simulink model "Autopilot_Controllers"  (R2020a)
settings: Solver=FixedStepAuto  StartTime=0.0  StopTime=10.0  FixedStep=0.01  RelTol=1e-3
model workspace: external: MAT-File E:\Autopilot\Task 7\GP04_Task7_Codes\JETSTAR_FC4_Parameters.mat (data not in the file)
values from neighbouring files (symbols this model uses):
  g = 32.17405    [JETSTAR_FC4_Parameters.mat]    (also in ReadExcelModified.m = aircraft_data(52))
  u_0 = 585.349466728    [JETSTAR_FC4_Parameters.mat]    (also in ReadExcelModified.m = s0(1))
settings Model: Creator=mohan  LastModifiedBy=mohan

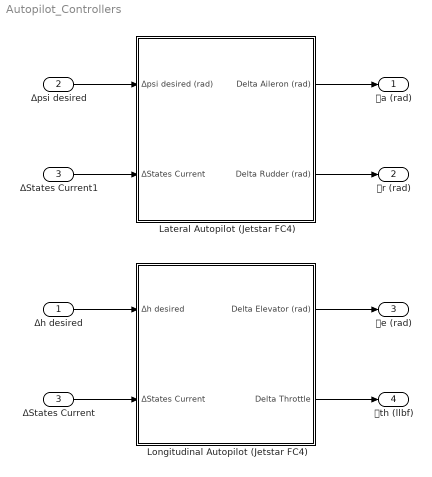
== system Autopilot_Controllers ==
  Δh desired : Inport
  Δpsi desired : Inport  Port=2
  ΔStates Current : Inport  Port=3
  Lateral Autopilot (Jetstar FC4) : Subsystem  mask{Kp_yaw=0.38326, taw_HPF=1/0.7, Kp_roll=1.0063, Kd_roll=0.32967, taw_coordination=20}
      mask prompts: Kp_yaw "Kp"; taw_HPF "Taw (Washout)"; Kp_roll "Kp"; Kd_roll "Kd"; taw_coordination "Taw"
      mask DialogControl ParameterGroupVar Prompt: Controllers
      mask DialogControl Container4 Prompt: Yaw Damper Gains (P + Washout)
      mask DialogControl Container5 Prompt: Roll Controller (PD)
      mask DialogControl Container6 Prompt: Coordinated Turn
  Longitudinal Autopilot (Jetstar FC4) : Subsystem  mask{Kp_alt=0.001862, Kd_alt=0.001694, Kp_pitch=1.6546, a_pitch=0.4868, Kd_pitch=0.52894, Kp_vel=1027.7, a_vel=0.05, Kd_vel=1523.9, zero_vel=0.1, pole_vel=0.7033}
      mask prompts: Kp_alt "Kp"; Kd_alt "Kd"; Kp_pitch "Kp"; a_pitch "a"; Kd_pitch "Kd"; Kp_vel "Kp"; a_vel "a"; Kd_vel "Kd"; zero_vel "Compensator Zero"; pole_vel "Compensator Pole"
      mask DialogControl ParameterGroupVar Prompt: Controllers
      mask DialogControl Container6 Prompt: Altitude Controller Gains (PID)
      mask DialogControl Container5 Prompt: Pitch Controller Gains (PID)
      mask DialogControl Container8 Prompt: Velocity Controller Gains (PI + Lead Compensator)
  ΔStates Current1 : InportShadow  Port=3
  𝛿a (rad) : Outport
  𝛿r (rad) : Outport  Port=2
  𝛿e (rad) : Outport  Port=3
  "𝛿th (llbf) " : Outport  Port=4
  wires:
  Δh desired/1 -> Longitudinal Autopilot (Jetstar FC4)/1(Δh desired)
  Δpsi desired/1 -> Lateral Autopilot (Jetstar FC4)/1(Δpsi desired (rad))
  ΔStates Current/1 -> Longitudinal Autopilot (Jetstar FC4)/2(ΔStates Current)
  ΔStates Current1/1 -> Lateral Autopilot (Jetstar FC4)/2(ΔStates Current)
  Longitudinal Autopilot (Jetstar FC4)/1(Delta Elevator (rad)) -> 𝛿e (rad)/1
  Longitudinal Autopilot (Jetstar FC4)/2(Delta Throttle) -> "𝛿th (llbf) "/1
  Lateral Autopilot (Jetstar FC4)/1(Delta Aileron (rad)) -> 𝛿a (rad)/1
  Lateral Autopilot (Jetstar FC4)/2(Delta Rudder (rad)) -> 𝛿r (rad)/1

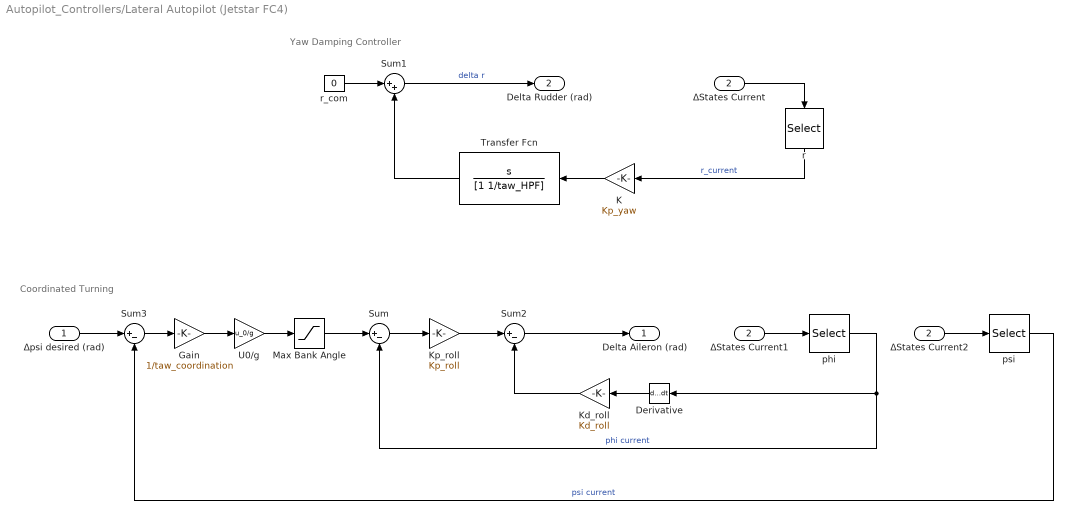
== system Autopilot_Controllers/Lateral Autopilot (Jetstar FC4) ==
  note: Coordinated Turning
  note: Yaw Damping Controller
  Δpsi desired (rad) : Inport
  ΔStates Current : Inport  Port=2
  Derivative : Derivative
  Gain : Gain  Gain=1/taw_coordination
  K : Gain  Gain=Kp_yaw
  Kd_roll : Gain  Gain=Kd_roll
  Kp_roll : Gain  Gain=Kp_roll
  Max Bank Angle : Saturate  UpperLimit=30*pi/180  LowerLimit=-30*pi/180
  Sum : Sum  Inputs=|+-
  Sum1 : Sum  Inputs=|++
  Sum2 : Sum  Inputs=|+-
  Sum3 : Sum  Inputs=|+-
  Transfer Fcn : TransferFcn  Numerator=[1 0]  Denominator=[1 1/taw_HPF]
  U0/g : Gain  Gain=u_0/g
  phi : Selector  InputPortWidth=15  IndexOptions=Index vector (dialog)  Indices=4  OutputSizes=1
  psi : Selector  InputPortWidth=15  IndexOptions=Index vector (dialog)  Indices=6  OutputSizes=1
  r : Selector  InputPortWidth=15  IndexOptions=Index vector (dialog)  Indices=12  OutputSizes=1
  r_com : Constant  Value=0
  ΔStates Current1 : InportShadow  Port=2
  ΔStates Current2 : InportShadow  Port=2
  Delta Aileron (rad) : Outport
  Delta Rudder (rad) : Outport  Port=2
  wires:
  r/1 -> K/1  "r_current"
  r_com/1 -> Sum1/1
  Transfer Fcn/1 -> Sum1/2
  K/1 -> Transfer Fcn/1
  Sum1/1 -> Delta Rudder (rad)/1  "delta r"
  ΔStates Current/1 -> r/1
  ΔStates Current1/1 -> phi/1
  Sum/1 -> Kp_roll/1
  Kd_roll/1 -> Sum2/2
  Sum2/1 -> Delta Aileron (rad)/1
  phi/1 -> Derivative/1, Sum/2  "phi current"
  Derivative/1 -> Kd_roll/1
  Kp_roll/1 -> Sum2/1
  Max Bank Angle/1 -> Sum/1
  Δpsi desired (rad)/1 -> Sum3/1
  ΔStates Current2/1 -> psi/1
  psi/1 -> Sum3/2  "psi current"
  Sum3/1 -> Gain/1
  Gain/1 -> U0/g/1
  U0/g/1 -> Max Bank Angle/1

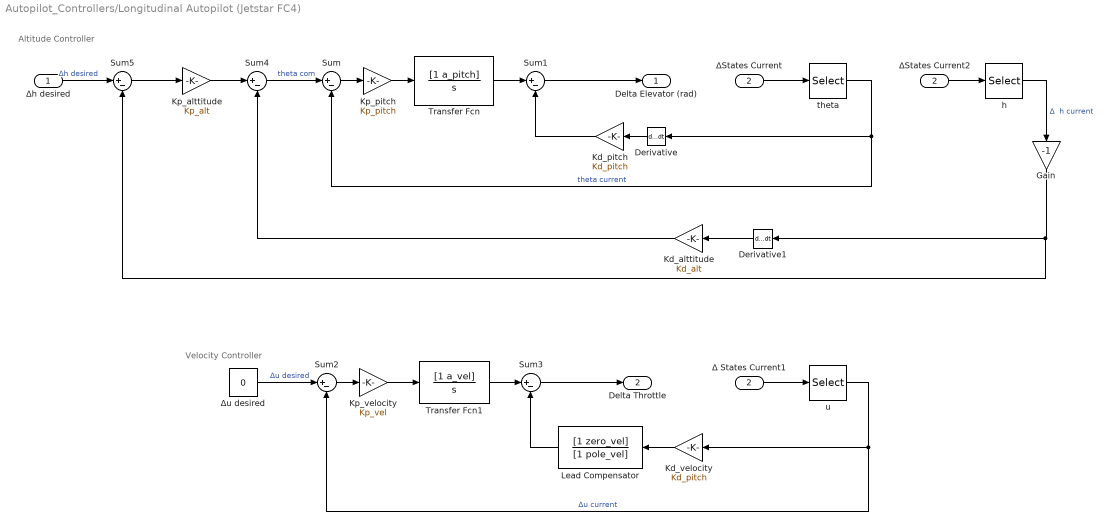
== system Autopilot_Controllers/Longitudinal Autopilot (Jetstar FC4) ==
  note: Velocity Controller
  note: Altitude Controller
  Δh desired : Inport
  ΔStates Current : Inport  Port=2
  Derivative : Derivative
  Derivative1 : Derivative
  Gain : Gain  Gain=-1
  Kd_alttitude : Gain  Gain=Kd_alt
  Kd_pitch : Gain  Gain=Kd_pitch
  Kd_velocity : Gain  Gain=Kd_pitch
  Kp_alttitude : Gain  Gain=Kp_alt
  Kp_pitch : Gain  Gain=Kp_pitch
  Kp_velocity : Gain  Gain=Kp_vel
  Lead Compensator : TransferFcn  Numerator=[1 zero_vel]  Denominator=[1 pole_vel]
  Sum{,1..5} (6 alike) : Sum  Inputs=|+-
  Transfer Fcn : TransferFcn  Numerator=[1 a_pitch]  Denominator=[1 0]
  Transfer Fcn1 : TransferFcn  Numerator=[1 a_vel]  Denominator=[1 0]
  h : Selector  InputPortWidth=15  IndexOptions=Index vector (dialog)  Indices=3  OutputSizes=1
  theta : Selector  InputPortWidth=15  IndexOptions=Index vector (dialog)  Indices=5  OutputSizes=1
  u : Selector  InputPortWidth=15  IndexOptions=Index vector (dialog)  Indices=7  OutputSizes=1
  Δ States Current1 : InportShadow  Port=2
  ΔStates Current2 : InportShadow  Port=2
  Δu desired : Constant  Value=0
  Delta Elevator (rad) : Outport
  Delta Throttle : Outport  Port=2
  wires:
  Transfer Fcn/1 -> Sum1/1
  ΔStates Current/1 -> theta/1
  Kp_pitch/1 -> Transfer Fcn/1
  Sum/1 -> Kp_pitch/1
  Kd_pitch/1 -> Sum1/2
  Derivative/1 -> Kd_pitch/1
  Sum1/1 -> Delta Elevator (rad)/1
  Transfer Fcn1/1 -> Sum3/1
  Sum2/1 -> Kp_velocity/1
  Δ States Current1/1 -> u/1
  Kp_velocity/1 -> Transfer Fcn1/1
  Kd_velocity/1 -> Lead Compensator/1
  Δu desired/1 -> Sum2/1  "Δu desired"
  Sum3/1 -> Delta Throttle/1
  Lead Compensator/1 -> Sum3/2
  theta/1 -> Derivative/1, Sum/2  "theta current"
  u/1 -> Kd_velocity/1, Sum2/2  "Δu current"
  Sum5/1 -> Kp_alttitude/1
  Kd_alttitude/1 -> Sum4/2
  ΔStates Current2/1 -> h/1
  h/1 -> Gain/1  "Δ  h current"
  Kp_alttitude/1 -> Sum4/1
  Derivative1/1 -> Kd_alttitude/1
  Gain/1 -> Derivative1/1, Sum5/2
  Δh desired/1 -> Sum5/1  "Δh desired"
  Sum4/1 -> Sum/1  "theta com"
